simulink library "Cust_Library_planarPKM"  (R2024a)
settings: Solver=VariableStepAuto  StartTime=0.0  StopTime=10.0  RelTol=1e-3
undefined symbols (not defined in the file): param
libraries: simulink x1
(part 1 of 2)
settings Model: Creator=Mohammad  LastModifiedBy=mohammad_admin
settings SolverCC: AlgebraicLoopSolver=TrustRegion
settings DebuggingCC: UnconnectedInputMsg=warning  UnconnectedOutputMsg=warning  UnconnectedLineMsg=warning
settings ModelReferenceCC: EnableRefExpFcnMdlSchedulingChecks=on
settings RTWCC: GPUComputeCapability=3.5  DLArmComputeVersion=19.05

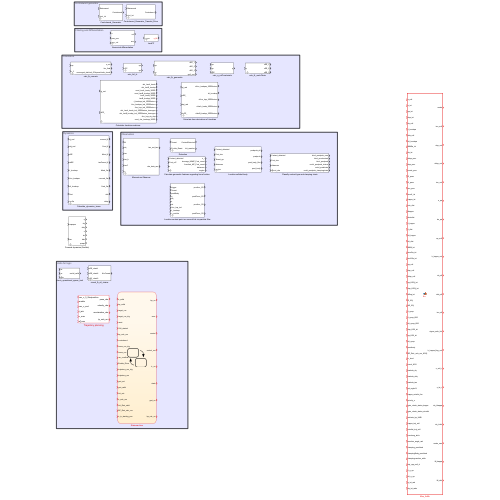
[thumbnail: Simulink's stored preview of the top-level diagram]
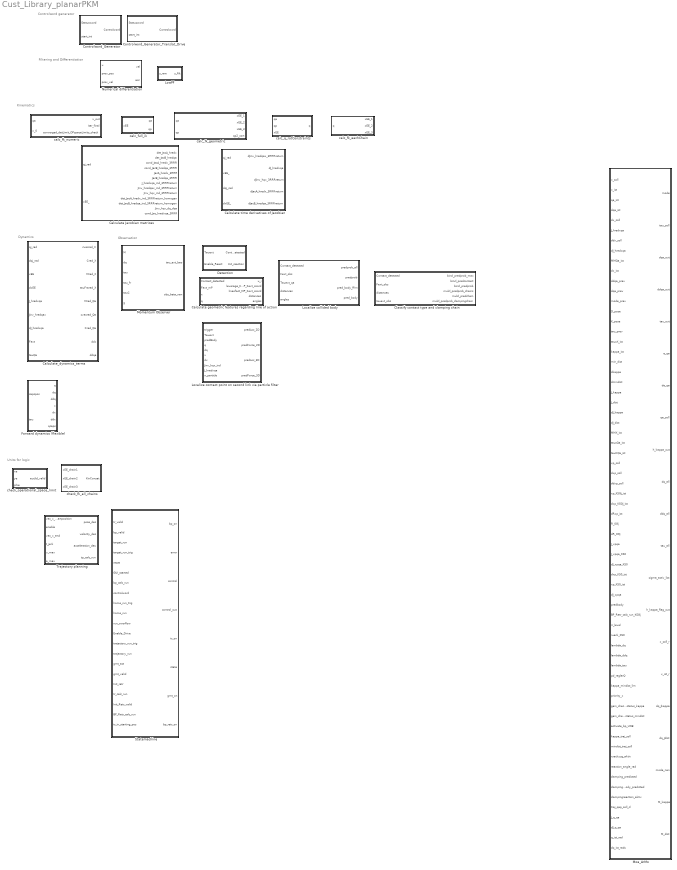
== system Cust_Library_planarPKM ==
  note: Units for logic
  note: Observation
  note: Dynamics
  note: Kinematics
  note: Filtering and Differentiation
  note: Controlword generator
  Calculate Jacobian matrices : Subsystem  mask(Calculate Jacobian matrices){l_all_id=param.l_all_id, r_fixPlat_j=param.r_fixPlat_j, r_mobPlat_j=param.r_mobPlat_j, psi_j=param.psi_j, beta_j=param.beta_j}
      mask prompts: l_all_id "l_all_id [m]"; r_fixPlat_j "r_fixPlat_j [m]"; r_mobPlat_j "r_mobPlat_j [m]"; psi_j "psi_j [rad]"; beta_j "beta_j [rad]"
      mask help: Function for determining the Jacobi matrices based on complete constraints h and reduced constraints hred
  Calculate geometric features regarding line of action : Subsystem  mask(Calculate geometric features regarding line of action){psi_j=param.psi_j, r_fixPlat_j=param.r_fixPlat_j, l_all_id=param.l_all_id}
      mask prompts: psi_j "psi_j [rad]"; r_fixPlat_j "r_fixPlat_j [m]"; l_all_id "l_all_id [m]"
  Calculate time derivatives of Jacobian : Subsystem  mask(Calculate time derivatives of Jacobian matrices){l_all=param.l_all, r_BasisPla_MobPla=param.r_BasisPla_MobPla}
      mask prompts: l_all "l_all [m]"; r_BasisPla_MobPla "r_BasisPla_MobPla [m]"
      mask help: Function for determining the time derivatives of the Jacobi matrices based on complete constraints h and reduced constraints hred
  Calculate_dynamics_terms : Subsystem  mask(Function for determining the dynamic terms){MDP=param.MDP, l_all=param.l_all, r_BasisPla_MobPla=param.r_BasisPla_MobPla}
      mask prompts: l_all "l_all [m]"; r_BasisPla_MobPla "r_BasisPla_MobPla [m]"
  Classify contact type and clamping chain : Subsystem  mask(Classify contact type and clamping chain){ffnn_clamping_param=param.ffnn_clamping_param, ffnn_clamping_chain_param=param.ffnn_clamping_chain_param}
  Controlword_Generator : Subsystem
      mask help: Initialization of the actuators using a controlword depending on the statusword and a user variable
      mask Help: Initialization of the actuators using a controlword depending on the statusword and a user variable
  Controlword_Generator_Translat_Drive : Subsystem  mask(Controlword generator for transl. drive){}
  Detection : Subsystem  mask(Function for determining whether a maximum permissible force, moment or torque value has been exceeded){ColDet_thresholds=param.CollDet_limit_MobPlat_soft}
  Forward dynamics (flexible) : Subsystem  mask(Forward dynamics with MuJoCo){capsule_active=param.capsule_active, t_sample=param.t_sample}
  Localize collided body : Subsystem  mask(Function for contact body classification with decision tree and fnn){min_dist_threshold=param.min_dist_threshold, min_angle_threshold_deg=param.min_angle_threshold_deg, min_torque_threshold=param.min_torque_threshold, ffnn_ClCollB_param=param.ffnn_ClCollB_param}
  Localize contact point on second link via particle filter : Subsystem  mask(Localize contact point on second link via particle filter){pf_dim=param.pf_dim, l_all=param.l_all, r_BasisPla_MobPla=param.r_BasisPla_MobPla, l_all_id=param.l_all_id, r_fixPlat_j=param.r_fixPlat_j, r_mobPlat_j=param.r_mobPlat_j, psi_j=param.psi_j, x_N_2D=param.x_N_2D, x_CovR_Inv_2D=param.x_CovR_Inv_2D, x_N_3D=param.x_N_3D, x_CovR_Inv_3D=param.x_CovR_Inv_3D}
      mask prompts: l_all "l_all [m]"; r_BasisPla_MobPla "r_BasisPla_MobPla [m]"; l_all_id "l_all_id [m]"; r_fixPlat_j "r_fixPlat_j [m]"; r_mobPlat_j "r_mobPlat_j [m]"; psi_j "psi_j [rad]"
  LowPF : Subsystem  mask(1st order low-pass filter){f_lp=param.f_lp_Hz, t_sample=param.t_sample, initial_value=zeros(1,1)}
      mask prompts: f_lp "f_lp [Hz]"; t_sample "t_sample [s]"
  Moe_ArMo : MATLAB Function  TreatAsAtomicUnit=on
  Momentum Observer : Subsystem  mask{Ko=param.Kox, t_sample=param.t_sample, initial_Fext=zeros(3,1)}
      mask prompts: Ko "Ko [1/s]"; t_sample "t_sample [s]"
  Numerical differentiation : Subsystem  mask(Function for numerical differentiation){t_sample=param.t_sample}
      mask prompts: t_sample "t_sample [s]"
      mask help: This function can be used to calculate the speed and acceleration of a variable u.
  Statemachine : Stateflow chart  TreatAsAtomicUnit=on
  Trajectory planning : Subsystem  mask(Function for calculating an online jerk-limited trajectory){}
  calc_fk_eachChain : Subsystem  mask(Function for determining the direct kinematics across all three leg chains){psi_j=param.psi_j, beta_j=param.beta_j, r_fixPlat_j=param.r_fixPlat_j, r_mobPlat_j=param.r_mobPlat_j, l_all_id=param.l_all_id}
  calc_fk_geometric : Subsystem  mask(Geometric forward kinematics){psi_j=param.psi_j, beta_j=param.beta_j, r_fixPlat_j=param.r_fixPlat_j, r_mobPlat_j=param.r_mobPlat_j, l_all_id=param.l_all_id}
      mask prompts: psi_j "psi_j [rad]"; beta_j "beta_j [rad]"; r_fixPlat_j "r_fixPlat_j [m]"; r_mobPlat_j "r_mobPlat_j [m]"; l_all_id "l_all_id [m]"
      mask help:
      | This function can be used to determine the platform positions over all three leg chains with known active and passive joint angles qa an qp.
      | In addition, the passive joint angle at the elbow is calculated with the defective incremental encoder.
  calc_fk_numeric : Subsystem  mask(Numeric forward kinematics){psi_j=param.psi_j, beta_j=param.beta_j, r_fixPlat_j=param.r_fixPlat_j, r_mobPlat_j=param.r_mobPlat_j, l_all_id=param.l_all_id, max_iter_find_fk_simulink=param.max_iter_find_fk_simulink, max_radius=param.max_radius, max_phie=param.max_phie, min_det_JacA_hredx=param.min_det_JacA_hredx, min_det_JacB_hredqa=param.min_det_JacB_hredqa}
      mask prompts: psi_j "psi_j [rad]"; beta_j "beta_j [rad]"; r_fixPlat_j "r_fixPlat_j [m]"; r_mobPlat_j "r_mobPlat_j [m]"; l_all_id "l_all_id [m]"; max_radius "max_radius [m]"; max_phie "max_phie [rad]"
      mask help:
      | Function for forward kinematics using Newton-Raphson
      | This function can be used to calculate the platform pose with known drive coordinates qa and an initial estimate x0.
  calc_full_ik : Subsystem  mask(Full inverse kinematics){psi_j=param.psi_j, beta_j=param.beta_j, r_fixPlat_j=param.r_fixPlat_j, r_mobPlat_j=param.r_mobPlat_j, l_all_id=param.l_all_id}
      mask prompts: psi_j "psi_j [rad]"; beta_j "beta_j [rad]"; r_fixPlat_j "r_fixPlat_j [m]"; r_mobPlat_j "r_mobPlat_j [m]"; l_all_id "l_all_id [m]"
      mask help:
      | Function for the complete geometric inverse kinematics
      | This function can be used to calculate the active and passive joint angles qa and qp for a known platform pose xEE.
  calc_q_rotConstraints : Subsystem  mask(Calculate q via rotational kinematic constraints){psi_j=param.psi_j}
      mask prompts: psi_j "psi_j [rad]"
  check_fk_all_chains : Subsystem  mask(Function for checking whether the direct kinematics of the three serial chains lead to the same platform pose){maxerrx=param.maxerrx, maxerry=param.maxerry}
  check_operational_space_limit : Subsystem  mask(Function for checking whether operational space limits are maintained){max_radius=param.max_radius, max_phie=param.max_phie}

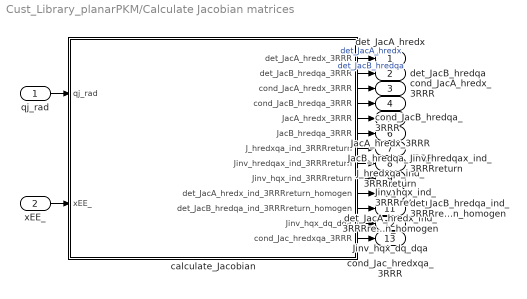
== system Cust_Library_planarPKM/Calculate Jacobian matrices ==
  qj_rad : Inport
  xEE_ : Inport  Port=2
  calculate_Jacobian : MATLAB Function  TreatAsAtomicUnit=on
  det_JacA_hredx : Outport
  det_JacB_hredqa : Outport  Port=2
  cond_JacA_hredx_3RRR : Outport  Port=3
  cond_JacB_hredqa_3RRR : Outport  Port=4
  JacA_hredx_3RRR : Outport  Port=5
  JacB_hredqa_3RRR : Outport  Port=6
  J_hredxqa_ind_3RRRreturn : Outport  Port=7
  Jinv_hredqax_ind_3RRRreturn : Outport  Port=8
  Jinv_hqx_ind_3RRRreturn : Outport  Port=9
  det_JacA_hredx_ind_3RRRreturn_homogen : Outport  Port=10
  det_JacB_hredqa_ind_3RRRreturn_homogen : Outport  Port=11
  Jinv_hqx_dq_dqa : Outport  Port=12
  cond_Jac_hredxqa_3RRR : Outport  Port=13
  wires:
  qj_rad/1 -> calculate_Jacobian/1(qj_rad)
  calculate_Jacobian/1(det_JacA_hredx_3RRR) -> det_JacA_hredx/1  "det_JacA_hredx"
  calculate_Jacobian/9(Jinv_hqx_ind_3RRRreturn) -> Jinv_hqx_ind_3RRRreturn/1
  xEE_/1 -> calculate_Jacobian/2(xEE_)
  calculate_Jacobian/5(JacA_hredx_3RRR) -> JacA_hredx_3RRR/1
  calculate_Jacobian/4(cond_JacB_hredqa_3RRR) -> cond_JacB_hredqa_3RRR/1
  calculate_Jacobian/7(J_hredxqa_ind_3RRRreturn) -> J_hredxqa_ind_3RRRreturn/1
  calculate_Jacobian/2(det_JacB_hredqa_3RRR) -> det_JacB_hredqa/1  "det_JacB_hredqa"
  calculate_Jacobian/3(cond_JacA_hredx_3RRR) -> cond_JacA_hredx_3RRR/1
  calculate_Jacobian/6(JacB_hredqa_3RRR) -> JacB_hredqa_3RRR/1
  calculate_Jacobian/8(Jinv_hredqax_ind_3RRRreturn) -> Jinv_hredqax_ind_3RRRreturn/1
  calculate_Jacobian/13(cond_Jac_hredxqa_3RRR) -> cond_Jac_hredxqa_3RRR/1
  calculate_Jacobian/10(det_JacA_hredx_ind_3RRRreturn_homogen) -> det_JacA_hredx_ind_3RRRreturn_homogen/1
  calculate_Jacobian/11(det_JacB_hredqa_ind_3RRRreturn_homogen) -> det_JacB_hredqa_ind_3RRRreturn_homogen/1
  calculate_Jacobian/12(Jinv_hqx_dq_dqa) -> Jinv_hqx_dq_dqa/1

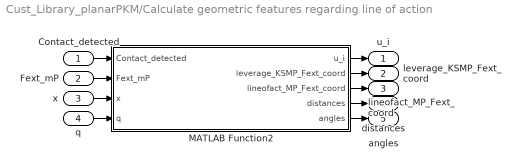
== system Cust_Library_planarPKM/Calculate geometric features regarding line of action ==
  Contact_detected : Inport
  Fext_mP : Inport  Port=2
  x : Inport  Port=3
  q : Inport  Port=4
  MATLAB Function2 : MATLAB Function  TreatAsAtomicUnit=on
  u_i : Outport
  leverage_KSMP_Fext_coord : Outport  Port=2
  lineofact_MP_Fext_coord : Outport  Port=3
  distances : Outport  Port=4
  angles : Outport  Port=5
  wires:
  MATLAB Function2/5(angles) -> angles/1
  MATLAB Function2/3(lineofact_MP_Fext_coord) -> lineofact_MP_Fext_coord/1
  MATLAB Function2/2(leverage_KSMP_Fext_coord) -> leverage_KSMP_Fext_coord/1
  Contact_detected/1 -> MATLAB Function2/1(Contact_detected)
  x/1 -> MATLAB Function2/3(x)
  MATLAB Function2/4(distances) -> distances/1
  Fext_mP/1 -> MATLAB Function2/2(Fext_mP)
  q/1 -> MATLAB Function2/4(q)
  MATLAB Function2/1(u_i) -> u_i/1

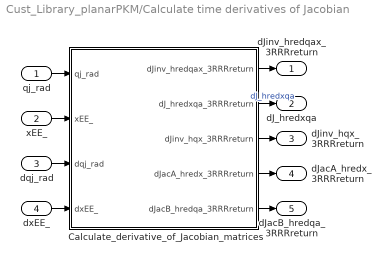
== system Cust_Library_planarPKM/Calculate time derivatives of Jacobian ==
  qj_rad : Inport
  xEE_ : Inport  Port=2
  dqj_rad : Inport  Port=3
  dxEE_ : Inport  Port=4
  Calculate_derivative_of_Jacobian_matrices : MATLAB Function  TreatAsAtomicUnit=on
  dJinv_hredqax_3RRRreturn : Outport
  dJ_hredxqa : Outport  Port=2
  dJinv_hqx_3RRRreturn : Outport  Port=3
  dJacA_hredx_3RRRreturn : Outport  Port=4
  dJacB_hredqa_3RRRreturn : Outport  Port=5
  wires:
  Calculate_derivative_of_Jacobian_matrices/4(dJacA_hredx_3RRRreturn) -> dJacA_hredx_3RRRreturn/1
  xEE_/1 -> Calculate_derivative_of_Jacobian_matrices/2(xEE_)
  dqj_rad/1 -> Calculate_derivative_of_Jacobian_matrices/3(dqj_rad)
  qj_rad/1 -> Calculate_derivative_of_Jacobian_matrices/1(qj_rad)
  Calculate_derivative_of_Jacobian_matrices/5(dJacB_hredqa_3RRRreturn) -> dJacB_hredqa_3RRRreturn/1
  Calculate_derivative_of_Jacobian_matrices/1(dJinv_hredqax_3RRRreturn) -> dJinv_hredqax_3RRRreturn/1
  Calculate_derivative_of_Jacobian_matrices/2(dJ_hredxqa_3RRRreturn) -> dJ_hredxqa/1  "dJ_hredxqa"
  dxEE_/1 -> Calculate_derivative_of_Jacobian_matrices/4(dxEE_)
  Calculate_derivative_of_Jacobian_matrices/3(dJinv_hqx_3RRRreturn) -> dJinv_hqx_3RRRreturn/1

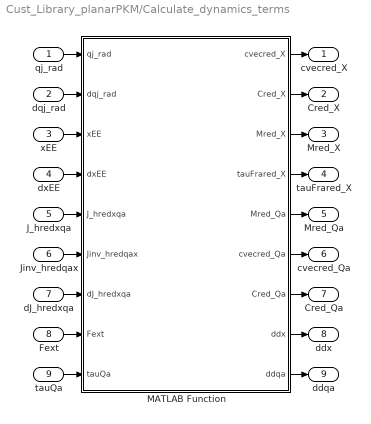
== system Cust_Library_planarPKM/Calculate_dynamics_terms ==
  qj_rad : Inport
  dqj_rad : Inport  Port=2
  xEE : Inport  Port=3
  dxEE : Inport  Port=4
  J_hredxqa : Inport  Port=5
  Jinv_hredqax : Inport  Port=6
  dJ_hredxqa : Inport  Port=7
  Fext : Inport  Port=8
  tauQa : Inport  Port=9
  MATLAB Function : MATLAB Function  TreatAsAtomicUnit=on
  cvecred_X : Outport
  Cred_X : Outport  Port=2
  Mred_X : Outport  Port=3
  tauFrared_X : Outport  Port=4
  Mred_Qa : Outport  Port=5
  cvecred_Qa : Outport  Port=6
  Cred_Qa : Outport  Port=7
  ddx : Outport  Port=8
  ddqa : Outport  Port=9
  wires:
  J_hredxqa/1 -> MATLAB Function/5(J_hredxqa)
  tauQa/1 -> MATLAB Function/9(tauQa)
  MATLAB Function/9(ddqa) -> ddqa/1
  MATLAB Function/4(tauFrared_X) -> tauFrared_X/1
  MATLAB Function/5(Mred_Qa) -> Mred_Qa/1
  xEE/1 -> MATLAB Function/3(xEE)
  MATLAB Function/6(cvecred_Qa) -> cvecred_Qa/1
  MATLAB Function/8(ddx) -> ddx/1
  Jinv_hredqax/1 -> MATLAB Function/6(Jinv_hredqax)
  dqj_rad/1 -> MATLAB Function/2(dqj_rad)
  dxEE/1 -> MATLAB Function/4(dxEE)
  dJ_hredxqa/1 -> MATLAB Function/7(dJ_hredxqa)
  Fext/1 -> MATLAB Function/8(Fext)
  MATLAB Function/2(Cred_X) -> Cred_X/1
  MATLAB Function/3(Mred_X) -> Mred_X/1
  qj_rad/1 -> MATLAB Function/1(qj_rad)
  MATLAB Function/1(cvecred_X) -> cvecred_X/1
  MATLAB Function/7(Cred_Qa) -> Cred_Qa/1

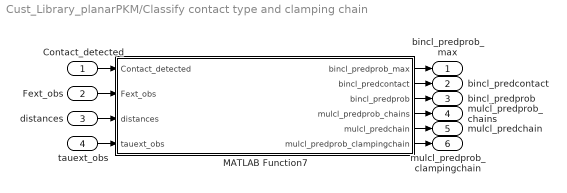
== system Cust_Library_planarPKM/Classify contact type and clamping chain ==
  Contact_detected : Inport
  Fext_obs : Inport  Port=2
  distances : Inport  Port=3
  tauext_obs : Inport  Port=4
  MATLAB Function7 : MATLAB Function  TreatAsAtomicUnit=on
  bincl_predprob_max : Outport
  bincl_predcontact : Outport  Port=2
  bincl_predprob : Outport  Port=3
  mulcl_predprob_chains : Outport  Port=4
  mulcl_predchain : Outport  Port=5
  mulcl_predprob_clampingchain : Outport  Port=6
  wires:
  MATLAB Function7/4(mulcl_predprob_chains) -> mulcl_predprob_chains/1
  distances/1 -> MATLAB Function7/3(distances)
  Fext_obs/1 -> MATLAB Function7/2(Fext_obs)
  Contact_detected/1 -> MATLAB Function7/1(Contact_detected)
  MATLAB Function7/1(bincl_predprob_max) -> bincl_predprob_max/1
  tauext_obs/1 -> MATLAB Function7/4(tauext_obs)
  MATLAB Function7/3(bincl_predprob) -> bincl_predprob/1
  MATLAB Function7/2(bincl_predcontact) -> bincl_predcontact/1
  MATLAB Function7/6(mulcl_predprob_clampingchain) -> mulcl_predprob_clampingchain/1
  MATLAB Function7/5(mulcl_predchain) -> mulcl_predchain/1

== system Cust_Library_planarPKM/Controlword_Generator ==
  Statusword : Inport
  start_int : Inport  Port=2
  StateMaschine StartUp - RotDrive 1 : Stateflow chart  TreatAsAtomicUnit=on
  Controlword : Outport
  wires:
  StateMaschine StartUp - RotDrive 1/1(Controlword) -> Controlword/1
  start_int/1 -> StateMaschine StartUp - RotDrive 1/2(start_int)
  Statusword/1 -> StateMaschine StartUp - RotDrive 1/1(Statusword)

== system Cust_Library_planarPKM/Controlword_Generator_Translat_Drive ==
  Statusword : Inport
  start_int : Inport  Port=2
  StateMaschine StartUp - TranslDrive1 : Stateflow chart  TreatAsAtomicUnit=on
  Controlword : Outport
  wires:
  StateMaschine StartUp - TranslDrive1/1(Controlword) -> Controlword/1
  Statusword/1 -> StateMaschine StartUp - TranslDrive1/1(Statusword)
  start_int/1 -> StateMaschine StartUp - TranslDrive1/2(start_int)

== system Cust_Library_planarPKM/Detection ==
  Tauext : Inport
  Enable_React : Inport  Port=2
  Detection : MATLAB Function  TreatAsAtomicUnit=on
  ContactDetected : Outport
  Init_reaction : Outport  Port=2
  wires:
  Tauext/1 -> Detection/1(Tauext)
  Detection/1(ContactDetected) -> ContactDetected/1
  Detection/2(init_reaction) -> Init_reaction/1
  Enable_React/1 -> Detection/2(collreact_enable)

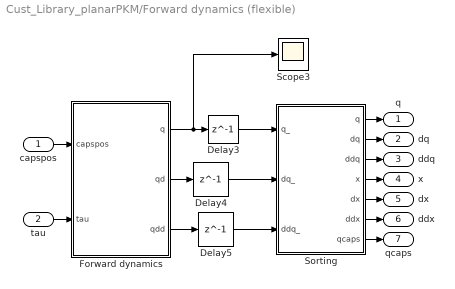
== system Cust_Library_planarPKM/Forward dynamics (flexible) ==
  capspos : Inport
  tau : Inport  Port=2
  Delay3 : Delay  DelayLength=1  InitialCondition=0
  Delay4 : Delay  DelayLength=1
  Delay5 : Delay  DelayLength=1
  Forward dynamics : MATLAB Function  TreatAsAtomicUnit=on
  Scope3 : Scope
  Sorting : MATLAB Function  TreatAsAtomicUnit=on
  q : Outport
  dq : Outport  Port=2
  ddq : Outport  Port=3
  x : Outport  Port=4
  dx : Outport  Port=5
  ddx : Outport  Port=6
  qcaps : Outport  Port=7
  wires:
  Forward dynamics/2(qd) -> Delay4/1
  Forward dynamics/1(q) -> Delay3/1, Scope3/1
  Delay4/1 -> Sorting/2(dq_)
  Delay3/1 -> Sorting/1(q_)
  tau/1 -> Forward dynamics/2(tau)
  Sorting/4(x) -> x/1
  Sorting/3(ddq) -> ddq/1
  Delay5/1 -> Sorting/3(ddq_)
  Sorting/5(dx) -> dx/1
  Forward dynamics/3(qdd) -> Delay5/1
  Sorting/7(qcaps) -> qcaps/1
  Sorting/6(ddx) -> ddx/1
  capspos/1 -> Forward dynamics/1(capspos)
  Sorting/2(dq) -> dq/1
  Sorting/1(q) -> q/1

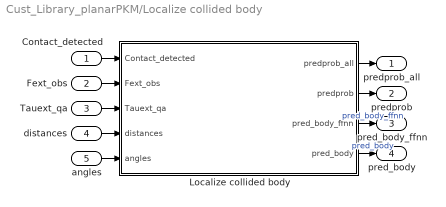
== system Cust_Library_planarPKM/Localize collided body ==
  Contact_detected : Inport
  Fext_obs : Inport  Port=2
  Tauext_qa : Inport  Port=3
  distances : Inport  Port=4
  angles : Inport  Port=5
  Localize collided body : MATLAB Function  TreatAsAtomicUnit=on
  predprob_all : Outport
  predprob : Outport  Port=2
  pred_body_ffnn : Outport  Port=3
  pred_body : Outport  Port=4
  wires:
  Tauext_qa/1 -> Localize collided body/3(Tauext_qa)
  Localize collided body/3(pred_body_ffnn) -> pred_body_ffnn/1  "pred_body_ffnn"
  distances/1 -> Localize collided body/4(distances)
  Fext_obs/1 -> Localize collided body/2(Fext_obs)
  Localize collided body/2(predprob) -> predprob/1
  Contact_detected/1 -> Localize collided body/1(Contact_detected)
  Localize collided body/1(predprob_all) -> predprob_all/1
  angles/1 -> Localize collided body/5(angles)
  Localize collided body/4(pred_body) -> pred_body/1  "pred_body"

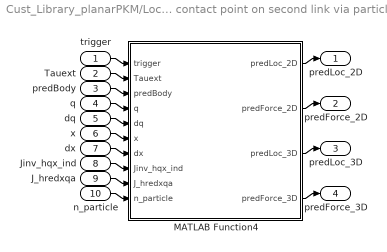
== system Cust_Library_planarPKM/Localize contact point on second link via particle filter ==
  trigger : Inport
  Tauext : Inport  Port=2
  predBody : Inport  Port=3
  q : Inport  Port=4
  dq : Inport  Port=5
  x : Inport  Port=6
  dx : Inport  Port=7
  Jinv_hqx_ind : Inport  Port=8
  J_hredxqa : Inport  Port=9
  n_particle : Inport  Port=10
  MATLAB Function4 : MATLAB Function  TreatAsAtomicUnit=on
  predLoc_2D : Outport
  predForce_2D : Outport  Port=2
  predLoc_3D : Outport  Port=3
  predForce_3D : Outport  Port=4
  wires:
  Jinv_hqx_ind/1 -> MATLAB Function4/8(Jinv_hqx_ind)
  MATLAB Function4/4(predForce_3D) -> predForce_3D/1
  dx/1 -> MATLAB Function4/7(dx)
  x/1 -> MATLAB Function4/6(x)
  n_particle/1 -> MATLAB Function4/10(n_particle)
  MATLAB Function4/2(predForce_2D) -> predForce_2D/1
  J_hredxqa/1 -> MATLAB Function4/9(J_hredxqa)
  q/1 -> MATLAB Function4/4(q)
  MATLAB Function4/1(predLoc_2D) -> predLoc_2D/1
  trigger/1 -> MATLAB Function4/1(trigger)
  predBody/1 -> MATLAB Function4/3(predBody)
  Tauext/1 -> MATLAB Function4/2(Tauext)
  dq/1 -> MATLAB Function4/5(dq)
  MATLAB Function4/3(predLoc_3D) -> predLoc_3D/1

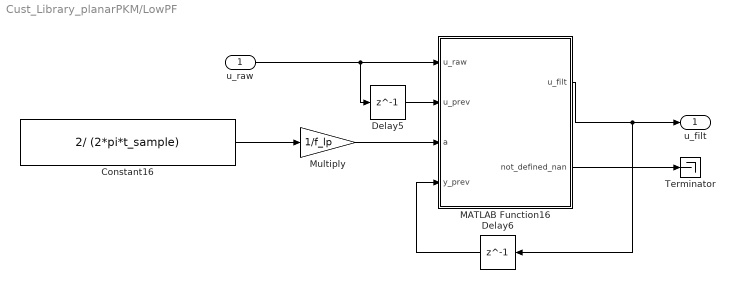
== system Cust_Library_planarPKM/LowPF ==
  u_raw : Inport
  Constant16 : Constant  Value=2/ (2*pi*t_sample)  SampleTime=-1
  Delay5 : Delay  DelayLength=1  InitialCondition=initial_value
  Delay6 : Delay  DelayLength=1  InitialCondition=initial_value
  MATLAB Function16 : MATLAB Function  TreatAsAtomicUnit=on
  Multiply : Gain  Gain=1/f_lp
  Terminator : Terminator
  u_filt : Outport
  wires:
  MATLAB Function16/2(not_defined_nan) -> Terminator/1
  Delay6/1 -> MATLAB Function16/4(y_prev)
  Constant16/1 -> Multiply/1
  MATLAB Function16/1(u_filt) -> Delay6/1, u_filt/1
  u_raw/1 -> MATLAB Function16/1(u_raw), Delay5/1
  Delay5/1 -> MATLAB Function16/2(u_prev)
  Multiply/1 -> MATLAB Function16/3(a)

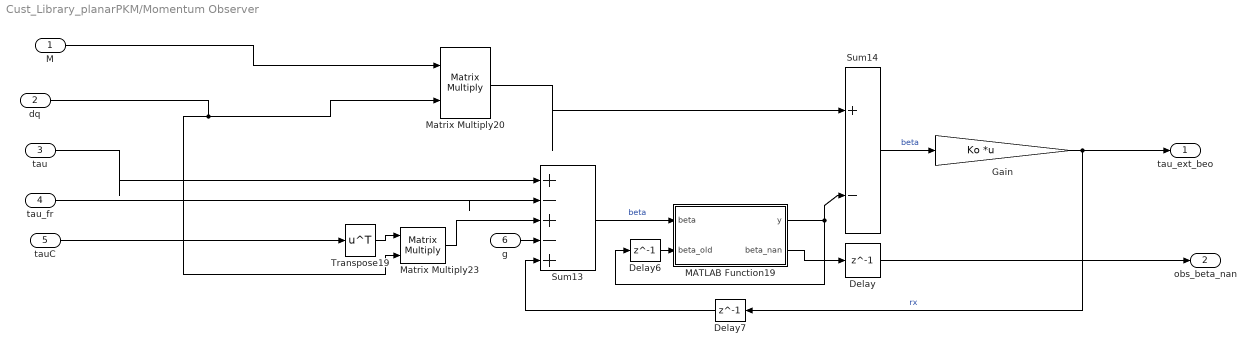
== system Cust_Library_planarPKM/Momentum Observer ==
  M : Inport
  dq : Inport  Port=2
  tau : Inport  Port=3
  tau_fr : Inport  Port=4
  tauC : Inport  Port=5
  g : Inport  Port=6
  Delay : Delay  DelayLength=1
  Delay6 : Delay  DelayLength=1  InitialCondition=initial_Fext
  Delay7 : Delay  DelayLength=1  InitialCondition=initial_Fext
  Gain : Gain  Gain=Ko  Multiplication=Matrix(K*u)
  MATLAB Function19 : MATLAB Function  TreatAsAtomicUnit=on
  Matrix Multiply20 : Product  Multiplication=Matrix(*)
  Matrix Multiply23 : Product  Multiplication=Matrix(*)
  Sum13 : Sum  Inputs=|+-+-+
  Sum14 : Sum  Inputs=|+-
  Transpose19 : Math  Operator=transpose  SignedPower=on
  tau_ext_beo : Outport
  obs_beta_nan : Outport  Port=2
  wires:
  Matrix Multiply23/1 -> Sum13/3
  MATLAB Function19/2(beta_nan) -> Delay/1
  Matrix Multiply20/1 -> Sum14/1
  dq/1 -> Matrix Multiply20/2, Matrix Multiply23/2
  Delay6/1 -> MATLAB Function19/2(beta_old)
  Sum14/1 -> Gain/1  "beta"
  tau_fr/1 -> Sum13/2
  Delay/1 -> obs_beta_nan/1
  Delay7/1 -> Sum13/5
  Transpose19/1 -> Matrix Multiply23/1
  Gain/1 -> tau_ext_beo/1, Delay7/1  "rx"
  Sum13/1 -> MATLAB Function19/1(beta)  "beta"
  MATLAB Function19/1(y) -> Sum14/2, Delay6/1
  tauC/1 -> Transpose19/1
  tau/1 -> Sum13/1
  M/1 -> Matrix Multiply20/1
  g/1 -> Sum13/4

== system Cust_Library_planarPKM/Numerical differentiation ==
  u : Inport
  prev_pos : Inport  Port=2
  prev_vel : Inport  Port=3
  MATLAB Function5 : MATLAB Function  TreatAsAtomicUnit=on
  vel : Outport
  acc : Outport  Port=2
  wires:
  u/1 -> MATLAB Function5/1(u)
  MATLAB Function5/1(vel) -> vel/1
  MATLAB Function5/2(acc) -> acc/1
  prev_pos/1 -> MATLAB Function5/2(prev_pos)
  prev_vel/1 -> MATLAB Function5/3(prev_vel)

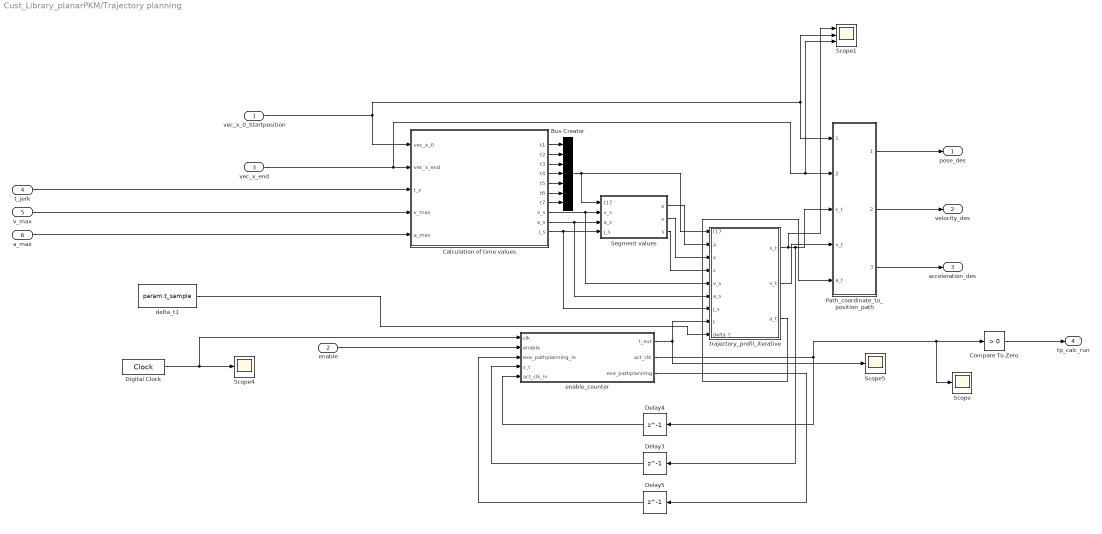
== system Cust_Library_planarPKM/Trajectory planning ==
  "vec_x_0_Startposition " : Inport
  enable : Inport  Port=2
  vec_x_end : Inport  Port=3
  t_jerk : Inport  Port=4
  v_max : Inport  Port=5
  a_max : Inport  Port=6
  Bus Creator : BusCreator  Inputs=7
  Calculation of time values : MATLAB Function  TreatAsAtomicUnit=on
  Compare To Zero : simulink/Logic and Bit Operations/Compare To Zero  relop=>  OutDataTypeStr=boolean
  Delay3 : Delay  DelayLength=1
  Delay4 : Delay  DelayLength=1
  Delay5 : Delay  DelayLength=1  InitialCondition=false
  Digital Clock : DigitalClock  SampleTime=param.t_sample
  Path_coordinate_to_position_path : MATLAB Function  TreatAsAtomicUnit=on
  Scope : Scope
  Scope1 : Scope  NumInputPorts=3
  Scope4 : Scope
  Scope5 : Scope
  Segment values : MATLAB Function  TreatAsAtomicUnit=on
  delta_t1 : Constant  Value=param.t_sample  SampleTime=param.t_sample
  enable_counter : MATLAB Function  TreatAsAtomicUnit=on
  "trajectory_profil_iterative " : MATLAB Function  TreatAsAtomicUnit=on
  pose_des : Outport  VectorParamsAs1DForOutWhenUnconnected=off
  velocity_des : Outport  Port=2  VectorParamsAs1DForOutWhenUnconnected=off
  acceleration_des : Outport  Port=3  VectorParamsAs1DForOutWhenUnconnected=off
  tp_calc_run : Outport  Port=4  VectorParamsAs1DForOutWhenUnconnected=off
  wires:
  enable/1 -> enable_counter/2(enable)
  vec_x_end/1 -> Calculation of time values/2(vec_x_end), Scope1/3, Path_coordinate_to_position_path/2(vec_x_end)
  Path_coordinate_to_position_path/3(vec_x_ddt) -> acceleration_des/1
  Path_coordinate_to_position_path/2(vec_x_dt) -> velocity_des/1
  t_jerk/1 -> Calculation of time values/3(t_v)
  Compare To Zero/1 -> tp_calc_run/1
  Path_coordinate_to_position_path/1(vec_x_t) -> pose_des/1
  a_max/1 -> Calculation of time values/5(a_max)
  v_max/1 -> Calculation of time values/4(v_max)
  Delay5/1 -> enable_counter/3(exe_pathplanning_in)
  enable_counter/3(exe_pathplanning) -> Delay5/1
  Delay4/1 -> enable_counter/5(act_clk_in)
  enable_counter/2(act_clk) -> Delay4/1, Compare To Zero/1, Scope/1
  enable_counter/1(t_out) -> Scope5/1, "trajectory_profil_iterative "/8(t)
  Delay3/1 -> enable_counter/4(s_t)
  Digital Clock/1 -> Scope4/1, enable_counter/1(clk)
  "trajectory_profil_iterative "/1(s_t) -> Scope1/1, Delay3/1, Path_coordinate_to_position_path/3(s_t)
  "trajectory_profil_iterative "/2(v_t) -> Path_coordinate_to_position_path/4(v_t)
  "trajectory_profil_iterative "/3(a_t) -> Path_coordinate_to_position_path/5(a_t)
  delta_t1/1 -> "trajectory_profil_iterative "/9(delta_t)
  Calculation of time values/5(t5) -> Bus Creator/5
  Segment values/2(v) -> "trajectory_profil_iterative "/3(v)
  Calculation of time values/10(j_s) -> Segment values/4(j_s), "trajectory_profil_iterative "/7(j_s)
  Calculation of time values/9(a_s) -> Segment values/3(a_s), "trajectory_profil_iterative "/6(a_s)
  Calculation of time values/3(t3) -> Bus Creator/3
  Calculation of time values/1(t1) -> Bus Creator/1
  Calculation of time values/8(v_s) -> Segment values/2(v_s), "trajectory_profil_iterative "/5(v_s)
  Calculation of time values/2(t2) -> Bus Creator/2
  Calculation of time values/4(t4) -> Bus Creator/4
  Segment values/3(s) -> "trajectory_profil_iterative "/4(s)
  Segment values/1(a) -> "trajectory_profil_iterative "/2(a)
  Calculation of time values/6(t6) -> Bus Creator/6
  Calculation of time values/7(t7) -> Bus Creator/7
  Bus Creator/1 -> "trajectory_profil_iterative "/1(t17), Segment values/1(t17)
  "vec_x_0_Startposition "/1 -> Calculation of time values/1(vec_x_0), Scope1/2, Path_coordinate_to_position_path/1(vec_x_0)

== system Cust_Library_planarPKM/calc_fk_eachChain ==
  q : Inport
  calc_fk_eachChain : MATLAB Function  TreatAsAtomicUnit=on
  xEE_1 : Outport
  xEE_2 : Outport  Port=2
  xEE_3 : Outport  Port=3
  wires:
  q/1 -> calc_fk_eachChain/1(q)
  calc_fk_eachChain/2(xEE_2) -> xEE_2/1
  calc_fk_eachChain/1(xEE_1) -> xEE_1/1
  calc_fk_eachChain/3(xEE_3) -> xEE_3/1

== system Cust_Library_planarPKM/calc_fk_geometric ==
  qa : Inport
  qp : Inport  Port=2
  Geometric forward kinematics : MATLAB Function  TreatAsAtomicUnit=on
  xEE_1 : Outport
  xEE_2 : Outport  Port=2
  xEE_3 : Outport  Port=3
  qp2_cort : Outport  Port=4
  wires:
  qa/1 -> Geometric forward kinematics/1(qa)
  Geometric forward kinematics/4(qp2_cort) -> qp2_cort/1
  qp/1 -> Geometric forward kinematics/2(qp)
  Geometric forward kinematics/2(xEE_2) -> xEE_2/1
  Geometric forward kinematics/3(xEE_3) -> xEE_3/1
  Geometric forward kinematics/1(xEE_1) -> xEE_1/1

== system Cust_Library_planarPKM/calc_fk_numeric ==
  qa : Inport
  x_0 : Inport  Port=2
  MATLAB Function1 : MATLAB Function  TreatAsAtomicUnit=on
  x_out : Outport
  iter_final : Outport  Port=2
  converged_detLimit_OPspaceLimits_check : Outport  Port=3
  wires:
  x_0/1 -> MATLAB Function1/2(x_0)
  MATLAB Function1/2(iter_final) -> iter_final/1
  MATLAB Function1/3(converged_detLimit_OPspaceLimits_check) -> converged_detLimit_OPspaceLimits_check/1
  MATLAB Function1/1(x_out) -> x_out/1
  qa/1 -> MATLAB Function1/1(qa)

== system Cust_Library_planarPKM/calc_full_ik ==
  xEE : Inport
  full_ik : MATLAB Function  TreatAsAtomicUnit=on
  qa : Outport
  qp : Outport  Port=2
  wires:
  full_ik/1(qa) -> qa/1
  xEE/1 -> full_ik/1(xEE)
  full_ik/2(qp) -> qp/1

== system Cust_Library_planarPKM/calc_q_rotConstraints ==
  qa : Inport
  qp : Inport  Port=2
  xEE : Inport  Port=3
  calc_q_rotConstraints : MATLAB Function  TreatAsAtomicUnit=on
  q : Outport
  wires:
  qa/1 -> calc_q_rotConstraints/1(qa)
  qp/1 -> calc_q_rotConstraints/2(qp)
  calc_q_rotConstraints/1(q) -> q/1
  xEE/1 -> calc_q_rotConstraints/3(xEE)

== system Cust_Library_planarPKM/check_fk_all_chains ==
  xEE_chain1 : Inport
  xEE_chain2 : Inport  Port=2
  xEE_chain3 : Inport  Port=3
  check_fk_all_chains : MATLAB Function  TreatAsAtomicUnit=on
  KinConsat : Outport
  wires:
  xEE_chain2/1 -> check_fk_all_chains/2(xEE_chain2)
  check_fk_all_chains/1(KinConsat) -> KinConsat/1
  xEE_chain3/1 -> check_fk_all_chains/3(xEE_chain3)
  xEE_chain1/1 -> check_fk_all_chains/1(xEE_chain1)

== system Cust_Library_planarPKM/check_operational_space_limit ==
  xe : Inport
  ye : Inport  Port=2
  phie : Inport  Port=3
  taskspace_limitation : MATLAB Function  TreatAsAtomicUnit=on
  euclid_valid : Outport
  wires:
  taskspace_limitation/1(euclid_valid) -> euclid_valid/1
  phie/1 -> taskspace_limitation/3(phie)
  ye/1 -> taskspace_limitation/2(ye)
  xe/1 -> taskspace_limitation/1(xe)

== matlab function Cust_Library_planarPKM/calc_fk_numeric/MATLAB Function1 ==
  data: qa input; x_out output; x_0 input; iter_final output; converged_detLimit_OPspaceLimits_check output; psi_j parameter; beta_j parameter; r_fixPlat_j parameter; r_mobPlat_j parameter; l_all_id parameter; max_iter_find_fk_simulink parameter; max_radius parameter; max_phie parameter; min_det_JacA_hredx parameter; min_det_JacB_hredqa parameter
function [x_out , iter_final, converged_detLimit_OPspaceLimits_check]= find_fk_simulink_(qa, x_0, psi_j, beta_j, r_fixPlat_j, r_mobPlat_j, l_all_id,...
                                  max_iter_find_fk_simulink, max_radius, max_phie, min_det_JacA_hredx, min_det_JacB_hredqa)

[x_out , iter_final, converged_detLimit_OPspaceLimits_check]= find_fk_simulink(qa, x_0, psi_j, beta_j, r_fixPlat_j, r_mobPlat_j, l_all_id,...
                                  max_iter_find_fk_simulink, max_radius, max_phie, min_det_JacA_hredx, min_det_JacB_hredqa);

== matlab function Cust_Library_planarPKM/Calculate geometric features regarding line of action/MATLAB Function2 ==
  data: Contact_detected input; Fext_mP input; u_i output; x input; q input; leverage_KSMP_Fext_coord output; lineofact_MP_Fext_coord output; distances output; angles output; psi_j parameter; r_fixPlat_j parameter; l_all_id parameter
function [u_i, leverage_KSMP_Fext_coord, lineofact_MP_Fext_coord, distances, angles] = CalcGeomFeatures_(Contact_detected, Fext_mP, x, q, psi_j, r_fixPlat_j, l_all_id)
    if Contact_detected
        [u_i, leverage_KSMP_Fext_coord, lineofact_MP_Fext_coord, distances, angles] = CalcGeomFeatures(Fext_mP, x, q, psi_j, r_fixPlat_j, l_all_id);
    else
        u_i = zeros(2,1);
        leverage_KSMP_Fext_coord = zeros(2,2);
        lineofact_MP_Fext_coord = zeros(2,2);
        distances = zeros(3,1);
        angles = zeros(3,1);
    end

== matlab function Cust_Library_planarPKM/calc_full_ik/full_ik ==
  data: xEE input; qa output; qp output; psi_j parameter; beta_j parameter; r_fixPlat_j parameter; r_mobPlat_j parameter; l_all_id parameter
function [qa, qp] = calcq_(xEE, psi_j, beta_j, r_fixPlat_j, r_mobPlat_j, l_all_id)
    [qa, qp] = calcq(xEE, psi_j, beta_j, r_fixPlat_j, r_mobPlat_j, l_all_id);
end

== matlab function Cust_Library_planarPKM/Forward dynamics (flexible)/Sorting ==
  data: q_ input; q output; dq_ input; ddq_ input; dq output; ddq output; x output; dx output; ddx output; qcaps output; capsule_active parameter
function [q, dq, ddq, x, dx, ddx, qcaps] = fcn(q_, dq_, ddq_, capsule_active)
    % Function for sorting the Mujoco sizes
    % Input:
    % q_ in m and rad: Vector of capsule, joint and platform coordinates (14x1)
    % qd_ in m/s and rad/s: Vector of capsule, joint and platform velocities (14x1)
    % qdd_ in m/s^2 and rad/s^2: Vector of capsule, joint and platform accelerations (14x1)
    %
    % Output:
    % q in rad: Vector of platform coordinates (9x1)
    % dq in rad/s: Vector of platform velocities (9x1)
    % ddq in rad/s^2: Vector of platform accelerations (9x1)
    % x in m and rad: Vector of platform coordinates (3x1)
    % dx in m/s and rad/s: Vector of platform velocities (3x1)
    % ddx in m/s^2 and rad/s^2: Vector of platform accelerations (3x1)
    % qcaps in m: vector of capsule coordinates (2x1)
    
    % Aran Mohammad, aran.mohammad@imes.uni-hannover.de, 2022-12
    % (C) Institute for Mechatronic Systems, Leibniz University Hanover
if capsule_active == 1
    qcaps = q_([1 2]) + [0.4; 0.3];
    q = q_([3 4 5 9 10 11 12 13 14]);
    x = q_([6 7 8]);
    
    dq = dq_([3 4 5 9 10 11 12 13 14]);
    dx = dq_([6 7 8]);
    
    ddq = ddq_([3 4 5 9 10 11 12 13 14]);
    ddx = ddq_([6 7 8]);
else
    qcaps = [0; 0];
    q = q_([1 2 3 7 8 9 10 11 12]);
    x = q_([4 5 6]);
    
    dq = dq_([1 2 3 7 8 9 10 11 12]);
    dx = dq_([4 5 6]);
    
    ddq = ddq_([1 2 3 7 8 9 10 11 12]);
    ddx = ddq_([4 5 6]);
end

== matlab function Cust_Library_planarPKM/Detection/Detection ==
  data: Tauext input; ColDet_thresholds parameter; ContactDetected output; init_reaction output; collreact_enable input
function [ContactDetected, init_reaction] = fcn(Tauext, ColDet_thresholds, collreact_enable)
    % Function for determining whether a maximum permissible force or torque value has been exceeded 
    % Input:
    % Fext_MobP in N and Nm: Estimated contact forces in platform coordinates (3x1)
    % ColDet_thresholds in N and Nm: Permissible maximum values (3x1)
    % colldect_enable: =1, activate this safety function (1x1)
    %
    % Output:
    % y: True, if exceeded (1x1)
    
    % Aran Mohammad, aran.mohammad@imes.uni-hannover.de, 2022-12
    % (C) Institute for Mechatronic Systems, Leibniz University Hanover
    
    if norm(Tauext(:))>1e-3 && (sum(abs(Tauext) >= ColDet_thresholds)>0)
        ContactDetected = true;
    else
        ContactDetected = false;
    end
    
    if collreact_enable && ContactDetected
        init_reaction = true;
    else
        init_reaction = false;
    end
end

== stateflow chart Cust_Library_planarPKM/Controlword_Generator/StateMaschine StartUp - RotDrive 1 ==
  state State0
    during:
    Controlword = 0;
  state State1
    during: Controlword = 0;
  state State2
    during: Controlword = 128;
  state State3
    during: Controlword = 2;
  state State4
    during: Controlword = 7;
  state State5
    during: Controlword = 15;
  (default) -> State0
  State5 -> State0 : [start_int == 0]
  State4 -> State0 [order 1] : [start_int == 0]
  State3 -> State0 [order 2] : [start_int == 0]
  State2 -> State0 [order 2] : [start_int == 0]
  State1 -> State0 [order 3] : [start_int == 0]
  State0 -> State1 : [ start_int == 1  ]
  State1 -> State3 [order 2] : [ Statusword == 4672 ]
  State1 -> State2 [order 1] : [ Statusword == 4648 ]
  State2 -> State3 [order 1] : [ Statusword == 4672 ]
  State3 -> State4 [order 1] : [ Statusword == 4609 ]
  State4 -> State5 [order 2] : [ Statusword == 4643 ]
  data: Statusword input; Controlword output; start_int input

== matlab function Cust_Library_planarPKM/calc_fk_geometric/Geometric forward kinematics ==
  data: qa input; qp input; xEE_1 output; xEE_2 output; xEE_3 output; qp2_cort output; psi_j parameter; beta_j parameter; r_fixPlat_j parameter; r_mobPlat_j parameter; l_all_id parameter
function [xEE_1, xEE_2, xEE_3, qp2_cort] = calcEE_qp2Corrected_return(qa, qp, psi_j, beta_j, r_fixPlat_j, r_mobPlat_j, l_all_id)
    [xEE_1, xEE_2, xEE_3, qp2_cort] = calcEE_qp2Corrected(qa, qp, psi_j, beta_j, r_fixPlat_j, r_mobPlat_j, l_all_id);
end

== matlab function Cust_Library_planarPKM/Trajectory planning/trajectory_profil_iterative  ==
  data: t17 input; a input; v input; s input; v_s input; s_t output; a_s input; j_s input; t input; delta_t input; v_t output; a_t output
function [s_t,v_t,a_t] = trajectory_profil_iterative(t17,a,v,s,v_s,a_s,j_s,t,delta_t)
%UNTITLED4 Summary of this function goes here
%   Detailed explanation goes here
    %t = step * delta_t;
    
    t2_ = t17(1) + t17(2);
    t3_ = t2_ + t17(3);
    t4_ = t3_ + t17(4);
    t5_ = t4_ + t17(5);
    t6_ = t5_ + t17(6);
    t7_ = t6_ + t17(7);
    
    if t < t17(1)
        a_t = j_s * t;
        v_t= 0.5 * j_s * t^2;
        s_t = (j_s/6)*t^3;
    elseif t < t2_
        t = t - t17(1);
        s_t = 0.5 * a_s * t^2 + v(1) * t + s(1);
        v_t = a_s * t + v(1);
        a_t = a_s;
    elseif t < t3_
        t = t - t2_;
        s_t = s(2) + 0.5*a(2)*t^2+  v(2) * t - (j_s/6)*t^3;
        v_t = v(2)  - 0.5*j_s*t^2+ a(2) * t;
        a_t = a(2) - j_s * t;
    elseif t < t4_
        t = t - t3_;
        s_t = s(3)  + v_s * t;
        v_t = v_s;
        a_t = 0;
    elseif t < t5_
        t = t - t4_;
        s_t  = s(4) + v(4) * t - (j_s/6) * t^3;
        v_t  = v(4) - 0.5*j_s*t^2;
        a_t  = -j_s * t;
    elseif t < t6_
        t = t - t5_;
        s_t   = -a_s * t^2 * 0.5 + v(5) * t + s(5);
        v_t   = -a_s * t       +  v(5);
        a_t   = -a_s; 
    elseif t < t7_
        t = t - t6_;
        s_t = 0.5 * a(6) * t^2 + (j_s/6) * t^3 + v(6) * t +s(6);
        v_t = a(6) * t + 0.5 * j_s * t^2 + v(6);
        a_t = a(6) + j_s * t;
    else
        s_t = 1.0;
        v_t = 0;
        a_t = 0;
    end
end

== matlab function Cust_Library_planarPKM/Trajectory planning/Path_coordinate_to_position_path ==
  data: vec_x_0 input; vec_x_t output; vec_x_end input; s_t input; v_t input; a_t input; vec_x_dt output; vec_x_ddt output
function [vec_x_t, vec_x_dt, vec_x_ddt] = fcn(vec_x_0, vec_x_end, s_t, v_t, a_t)
%#codegen
    vec_x_t = (vec_x_0 + s_t * (vec_x_end - vec_x_0));
    vec_x_dt = v_t * ((vec_x_end - vec_x_0));
    vec_x_ddt = a_t * ((vec_x_end - vec_x_0));
    
end

== matlab function Cust_Library_planarPKM/Trajectory planning/Calculation of time values ==
  data: vec_x_0 input; t1 output; vec_x_end input; t_v input; v_max input; a_max input; t2 output; t3 output; t4 output; t5 output; t6 output; t7 output; v_s output; a_s output; j_s output
function [t1,t2,t3,t4,t5,t6,t7,v_s,a_s,j_s] = Time_calculation(vec_x_0,vec_x_end,t_v,v_max,a_max)
%UNTITLED2 Summary of this function goes here
%   Detailed explanation goes here
    eps = 10^-6;
    delta_vec_x = vec_x_end - vec_x_0;
    s_end = max(abs(delta_vec_x));
    v_s  = v_max / s_end;
    a_s = a_max / s_end;
    j = a_max / t_v;
    j_s = j / s_end;
    
    %++++++++++
    % Bereich 1
    t_1a = a_s / j_s;           % Wird a_max_s erreicht?
    t_1v = sqrt(v_s / j_s);     % Wird v_max_s erreicht?
    t_1s = (1/(2*j_s))^(1/3);   % Wird s_e erreicht?
    t1 = min([t_1a, t_1v, t_1s]);
    
    % Berechnen von Beschl., Geschw. und zurückgelegter Strecke nach 
    % Abschnitt 1.
    a_prv = j_s * t1;
    v_prv = 0.5 * j_s * t1^2;
    s_prv = (j_s/6)*t1^3;
    t_prv = t1;
 
    %++++++++++
    % Bereich 2
    % Wird nur erreicht, wenn a_max (a_s) erreicht wurde.
    if abs(a_prv - a_s) < eps
        t_2v    = (v_s -a_s*t_prv) / a_s;
        t_2s    = -1.5*(a_s/j_s) + sqrt(0.25*(a_s/j_s)^2 + 1/a_s);
        % Abfangen negativer Zeiten.
        if t_2v < 0 || t_2s < 0
            if t_2v < 0 && t_2s < 0
                t2 = 0;
            elseif t_2v < 0 
                t2 = t_2s;
            elseif t_2s < 0
                t2 = t_2v;
            else
                t2 = 0;
                %disp('[ERROR] In Berechnung der Eckzeiten, Bereich 2');
            end
        else
            t2 = min(t_2v,t_2s);
        end
        
        % Berechnen von Beschl., Geschw. und zurückgelegter Strecke nach 
        % Abschnitt 2.
        if t2 > 0
            s_prv = 0.5 * a_s * t2^2 + v_prv * t2 + s_prv;
            v_prv = a_s * t2 + v_prv;
            a_prv = a_s;
        end
    else
        %disp('Bereich 2 wird übersprungen');
        t2 = 0;
    end

    %++++++++++
    % Bereich 3
    % Wird immer erreicht
    t3    = a_prv / j_s;
    s_prv =  s_prv + 0.5*a_prv*t3^2+  v_prv * t3 - (j_s/6)*t3^3;
    v_prv = v_prv  - 0.5*j_s*t3^2+ a_prv * t3;
    a_prv = a_prv - j_s * t3;
    
    % +++++++++
    % Bereich 4
    % Wird nur erreicht, wenn v_max (v_s) erreicht wurde.
    if abs(v_prv - v_s) < eps
        t4 = (1-2*s_prv)/v_s;
        if t4 < 0
            %%disp('[ERROR] Funktion Zeitberechnung in Bereich 4');
            %disp('Zeit t4 ist negativ');
            t4 = 0;
        else
            s_prv = s_prv  + v_s * t4;
            v_prv = v_s;
            a_prv = 0;
        end
    else
        %disp('Bereich 4 wird übersprungen');
        t4 = 0;
    end
    % +++++++++
    % Bereich 5
    t5 = t1;
    s_prv  = s_prv + v_prv * t5 - (j_s/6) * t5^3;
    v_prv  =  v_prv - 0.5*j_s*t5^2;
    a_prv  = -j_s * t5;

    % +++++++++
    % Bereich 6
    t6 = t2;
    if t2 > 0
        s_prv   = -a_s * t6.^2 * 0.5 +  v_prv * t6 + s_prv;
        v_prv   = -a_s * t6          +  v_prv;
        a_prv   = -a_s; 
    else
        %disp('Bereich 6 wird übersprungen');
        t6 = 0;
    end
    
    % +++++++++
    % Bereich 7
    t7 = t1;
    s_prv = 0.5 * a_prv * t7^2 + (j_s/6) * t7^3 + v_prv * t7 +s_prv;
    
    % ++++++++
    % Plausibilitätsprüfung
     if abs(s_prv - 1.0) > eps
        %disp('s(t_end) ist nicht 1, sondern:');
        %disp(s_prv);
    end
    if (t1<0)||t2<0||(t3<0)||(t4<0)||(t5<0)||(t6< 0)||(t7<0)
        %disp('[ERROR] Plausibilitätsprüfung in Zeitberechnung');
        %disp('Grrr, irgendwas lief hier ganz schief');
    end    
end

== matlab function Cust_Library_planarPKM/Trajectory planning/enable_counter ==
  data: clk input; t_out output; enable input; exe_pathplanning_in input; s_t input; act_clk output; exe_pathplanning output; act_clk_in input
function [t_out, act_clk, exe_pathplanning] = fcn(clk, enable, exe_pathplanning_in,s_t,act_clk_in)
%#codegen
    if exe_pathplanning_in && s_t < 1
        t_out = clk - act_clk_in;
         exe_pathplanning = exe_pathplanning_in;
         act_clk = act_clk_in;
    else
        t_out = 0;
        exe_pathplanning = 0;
        act_clk = 0;
    end 

    if enable && ~exe_pathplanning_in
        act_clk = clk;
        exe_pathplanning = 1;
    end
    
   
end

== matlab function Cust_Library_planarPKM/Trajectory planning/Segment values ==
  data: t17 input; v_s input; a_s input; a output; j_s input; v output; s output
function [ a,v,s ] = Segment_values( t17,v_s,a_s,j_s )
%UNTITLED6 Summary of this function goes here
%   Detailed explanation goes here

    t1 = t17(1);
    t2 = t17(2);
    t3 = t17(3);
    t4 = t17(4);
    t5 = t17(5);
    t6 = t17(6);
    a_1 = j_s * t1;
    v_1 = 0.5 * j_s * t1^2;
    s_1 = (j_s/6)*t1^3;

    if t2 == 0
        s_2 = s_1;
        v_2 = v_1;
        a_2 = a_1;
    else
        s_2 = 0.5 * a_s * t2^2 + v_1 * t2 + s_1;
        v_2 = a_s * t2 + v_1;
        a_2 = a_s;
    end
    
    s_3 =  s_2 + 0.5*a_2*t3^2+  v_2 * t3 - (j_s/6)*t3^3;
    v_3 =  v_2 - 0.5*j_s*t3^2+ a_2 * t3;
    a_3 =  a_2 - j_s * t3;

    if t4 == 0
        s_4 = s_3;
        v_4 = v_3;
        a_4 = a_3;
    else
        s_4 = s_3  + v_s * t4;
        v_4 = v_s;
        a_4 = 0;
    end

    s_5  = s_4 + v_4 * t5 - (j_s/6) * t5^3;
    v_5  = v_4 - 0.5*j_s*t5^2;
    a_5  = -j_s * t5;

    if t6 == 0
        s_6 = s_5;
        v_6 = v_5;
        a_6 = a_5;
    else
        s_6   = -a_s * t6.^2 * 0.5 +  v_5 * t6 + s_5;
        v_6   = -a_s * t6          +  v_5;
        a_6   = -a_s; 
    end

    a = [a_1,a_2,a_3,a_4,a_5,a_6];
    v = [v_1,v_2,v_3,v_4,v_5,v_6];
    s = [s_1,s_2,s_3,s_4,s_5,s_6];
    

end

== matlab function Cust_Library_planarPKM/calc_fk_eachChain/calc_fk_eachChain ==
  data: q input; xEE_1 output; xEE_2 output; xEE_3 output; psi_j parameter; beta_j parameter; r_fixPlat_j parameter; r_mobPlat_j parameter; l_all_id parameter
function [xEE_1, xEE_2, xEE_3] = calcEE_eachChain_return(q, psi_j, beta_j, r_fixPlat_j, r_mobPlat_j, l_all_id)
    [xEE_1, xEE_2, xEE_3] = calcEE_eachChain(q, psi_j, beta_j, r_fixPlat_j, r_mobPlat_j, l_all_id);
end

== matlab function Cust_Library_planarPKM/Forward dynamics (flexible)/Forward dynamics ==
  data: capspos input; tau input; q output size=[14,1]; qd output; qdd output; capsule_active parameter; t_sample parameter
function [q, qd, qdd] = call_mujoco(capspos, tau, capsule_active, t_sample)
    % Function for the Mujoco call and output of the kinematic variables
    % Input:
    % capspos in m and m/s: Cap position and speed [posx velx posy vely] (4x1)
    % tau in Nm: Drive torques in drive coordinates (3x1)
    %
    % Output:
    % q_ in m and rad: Vector of capsule, joint and platform coordinates (14x1)
    % qd_ in m/s and rad/s: Vector of capsule, joint and platform velocities (14x1)
    % qdd_ in m/s^2 and rad/s^2: Vector of capsule, joint and platform accelerations (14x1)
    
    % Aran Mohammad, aran.mohammad@imes.uni-hannover.de, 2022-12
    % (C) Institute for Mechatronic Systems, Leibniz University Hanover

%#codegen
coder.extrinsic('mjx');
coder.extrinsic('evalin');
if capsule_active == 1
    mjx('set', 'ctrl', [capspos' tau']);
    mjx('step', t_sample/0.001);
    
    q_ = zeros(14,1); 
    qd = zeros(14,1); 
    qdd = zeros(14,1);    
    
    qoffset =[0.4; 0.3;
         25.5184; 122.3049; -237.8233; ...
         0; 0; 0; ...
         25.9632; 121.7747; -358.5010; ...
         24.3787; 124.6086; -479.4775]*pi/180;
else
    mjx('set', 'ctrl', tau');
    mjx('step', t_sample/0.001);

    q_woCapsule = zeros(12,1); 
    qd_woCapsule = zeros(12,1); 
    qdd_woCapsule = zeros(12,1);
    
    qoffset =[25.5184; 122.3049; -237.8233; ...
         0; 0; 0; ...
         25.9632; 121.7747; -358.5010; ...
         24.3787; 124.6086; -479.4775]*pi/180;
end
if capsule_active == 1
    q_ = mjx('get', 'qpos');
    q = q_ + qoffset;
else
    q_woCapsule = mjx('get', 'qpos');
    q = q_woCapsule + qoffset;
end
qd = mjx('get', 'qvel');
qdd = mjx('get', 'qacc');

== matlab function Cust_Library_planarPKM/check_fk_all_chains/check_fk_all_chains ==
  data: xEE_chain1 input; xEE_chain2 input; KinConsat output; xEE_chain3 input; maxerrx parameter; maxerry parameter
function KinConsat = checkKinCons_return(xEE_chain1, xEE_chain2, xEE_chain3, maxerrx, maxerry)
    KinConsat = checkKinCons(xEE_chain1, xEE_chain2, xEE_chain3, maxerrx, maxerry); 
end

== matlab function Cust_Library_planarPKM/Numerical differentiation/MATLAB Function5 ==
  data: u input; vel output; prev_pos input; prev_vel input; acc output; t_sample parameter
function [vel, acc] = fcn(u, prev_pos, prev_vel, t_sample)
    % Function for numerical differentiation
    % This function can be used to calculate the speed and acceleration of a variable u.
    % Input:
    % u: Angle/distance 
    % prev_pos: Previous angle/distance
    % prev_vel: Previous speed
    %
    % output:
    % vel: Numerically differentiated determined velocity
    % acc: Acceleration determined numerically differentiated
    
    % Aran Mohammad, aran.mohammad@imes.uni-hannover.de, 2022-12
    % (C) Institute for Mechatronic Systems, Leibniz University Hanover

    vel = (u-prev_pos)/t_sample;
    acc = (vel-prev_vel)/t_sample;

== matlab function Cust_Library_planarPKM/check_operational_space_limit/taskspace_limitation ==
  data: xe input; euclid_valid output; ye input; phie input; max_radius parameter; max_phie parameter
function euclid_valid = fcn(xe,ye, phie, max_radius, max_phie)
    % Function for checking whether operational space limits are maintained
    % Input:
    % xe in m: Platform position in the x-axis CS0 (1x1)
    % ye in m: Platform position in the y-axis CS0(1x1)
    % phie in rad: Platform orientation around the z-axis CS0(1x1)
    %
    % Output:
    % euclid_valid: =1, if workspace limits are fulfilled (1x1)
    
r = sqrt(xe^2+ye^2);

if r <= max_radius && abs(phie)< max_phie
    euclid_valid = true;
else
    euclid_valid = false;
end

== stateflow chart Cust_Library_planarPKM/Controlword_Generator_Translat_Drive/StateMaschine StartUp - TranslDrive1 ==
  state State0
    during:
    Controlword = 0;
  note: Notation ist:
      | Zustand: Definition
      | SW als Bedingung
      | CW als Ausgabe, solange Bedingung erfüllt
      |
      | State0: start is not set
      | CW=0
      |
      | State1: start is set / Nicht Einschaltbereit / Not Ready to Switch On
      | start_int=1
      | CW=0
      |
      | State2: Reset Störung
      | SW=40=0101000 : Schnellhalt, Störung
      | CW=128=10000000 : Reset Störung
      |
      | State3: Stillsetzen, sobald Slave sagt "Einschaltsperre/Switch On Disabled"
      | SW=37984=37888+96=1001010001100000 : Einschaltsperre, Schnellhalt
      | CW=6=00000110 : Schnellhalt, Spannung sperren
      |
      | State4: Einschalten, sobald Slave sagt "Einschaltbereit / Ready to switch on"
      | SW=37921=37888+33= 1001010000100001 : Schnellhalt, Einschaltbereit
      | CW=7=00000111 : Schnellhalt, Spannung sperren, Spannung sperren
      |
      | State5:  Betrieb freigeben, sobald Slave sagt "Eingeschaltet / Switched On"
      | SW=37923=37888+35=1001010000100011 : Einschaltbereit, Eingeschaltet, Schnellhalt
      | CW=15=00001111 : Betrieb freigegeben, Schnellhalt, Spannung sperren, Einschalten
      |
      | State6: Slave sagt "Betrieb freigegeben / Operation enabled" und deswegen ist der State nicht hier abgebildet
      | SW=37927+37888+39=1001010000100111 : Schnellhalt, Betrieb freigegeben, Eingeschaltet, Einschaltbereit
  state State1
    during: Controlword = 0;
  state State2
    during: Controlword = 128;
  state State3
    during: Controlword = 6;
  state State4
    during: Controlword = 7;
  state State5
    during: Controlword = 15;
  (default) -> State0
  State5 -> State0 : [start_int == 0]
  State4 -> State0 [order 1] : [start_int == 0]
  State3 -> State0 [order 2] : [start_int == 0]
  State2 -> State0 [order 2] : [start_int == 0]
  State1 -> State0 [order 3] : [start_int == 0]
  State0 -> State1 : [ start_int == 1  ]
  State1 -> State3 [order 2] : [ Statusword == 37984 || Statusword == 38000]
  State1 -> State2 [order 1] : [ Statusword == 37896 ]
  State2 -> State3 [order 1] : [ Statusword == 37984 ]
  State3 -> State4 [order 1] : [ Statusword == 37937 ]
  State4 -> State5 [order 2] : [ Statusword == 37939 ]
  data: Statusword input; Controlword output; start_int input

== matlab function Cust_Library_planarPKM/Momentum Observer/MATLAB Function19 ==
  data: beta input; y output; beta_old input; t_sample parameter; beta_nan output
function [y, beta_nan] =intu (beta, beta_old, t_sample)

y_ = beta_old + t_sample*beta; 

if sum(isnan(y_))
    y = zeros(3,1);
    beta_nan = true;
else
    y = y_;    
    beta_nan = false;
end
